simulink model "model1"  (R2021b)
settings: Solver=VariableStepAuto  StartTime=0.0  StopTime=10.0  RelTol=1e-3
values from neighbouring files (symbols this model uses):
  A = [   0    1 ... (first row only)    [config.m]
  A_m = [     0      1 ... (first row only)    [config.m]
  b = [0 ... (first row only)    [config.m]
  b_m = [0 ... (first row only)    [config.m]
  disturbance = 0    [config.m]    (also in task1.m = 1; task2.m = 1)
  gamma = 10000    [task1.m]    (also in task2.m = 100)
  k = b_0/a_m_0    (= 0.0434782608696)    [config.m]
  P = lyap(A_m', Q)    [config.m]
  x_0 = [1; 0]    [config.m]
settings Model: LastModifiedBy=popov
settings OptimizationCC: BlockReduction=off  BooleanDataType=off
settings DebuggingCC: SaveWithParameterizedLinksMsg=none  UnderspecifiedInitializationDetection=Classic  MergeDetectMultiDrivingBlocksExec=none  SignalResolutionControl=TryResolveAllWithWarning
settings HardwareCC: TargetUnknown=on
settings ModelReferenceCC: PropagateSignalLabelsOutOfModel=off

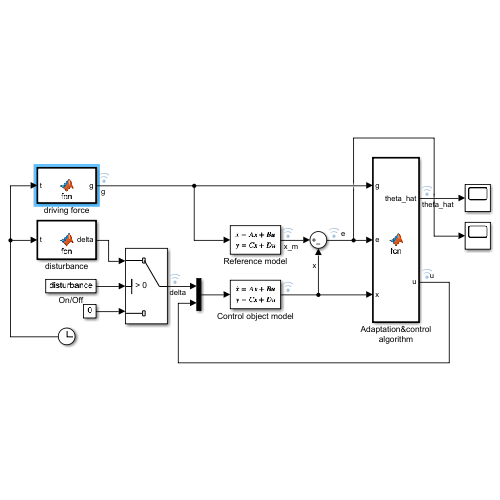
[thumbnail: Simulink's stored preview of the top-level diagram]
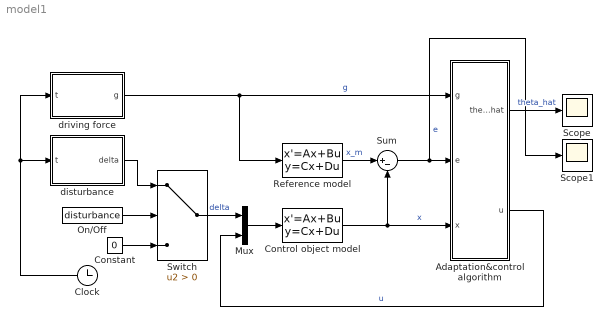
== system model1 ==
  Adaptation&control algorithm : MATLAB Function  TreatAsAtomicUnit=on
  Clock : Clock
  Constant : Constant  Value=0
  Control object model : StateSpace  A=A  B=[eye(2) b]  C=eye(2)  D=zeros(2,3)  InitialCondition=x_0
  Mux : Mux  Inputs=2
  On/Off : Constant  Value=disturbance
  Reference model : StateSpace  A=A_m  B=b_m  C=eye(2)  D=[0;0]  InitialCondition=0
  Scope : Scope
  Scope1 : Scope
  Sum : Sum  Inputs=|+-
  Switch : Switch  Criteria=u2 > Threshold
  disturbance : MATLAB Function  TreatAsAtomicUnit=on
  driving force : MATLAB Function  TreatAsAtomicUnit=on
  wires:
  Clock/1 -> disturbance/1(t), driving force/1(t)
  driving force/1(g) -> Reference model/1, Adaptation&control algorithm/1(g)  "g"
  Control object model/1 -> Sum/2, Adaptation&control algorithm/3(x)  "x"
  Sum/1 -> Scope1/1, Adaptation&control algorithm/2(e)  "e"
  Adaptation&control algorithm/2(u) -> Mux/2  "u"
  Reference model/1 -> Sum/1  "x_m"
  Mux/1 -> Control object model/1
  disturbance/1(delta) -> Switch/1
  Adaptation&control algorithm/1(theta_hat) -> Scope/1  "theta_hat"
  Constant/1 -> Switch/3
  Switch/1 -> Mux/1  "delta"
  On/Off/1 -> Switch/2

== matlab function model1/driving force ==
  data: t input; g output
function g = fcn(t)

g = 2*sign(sin(0.4*t)) + 3;

== matlab function model1/disturbance ==
  data: t input; delta output
function delta = fcn(t)

delta = [0.6*sin(10*t) + 0.1*sin(50*t);
        0.5*cos(12*t) + 0.2*sin(30*t)];

== matlab function model1/Adaptation&control algorithm ==
  data: theta_hat output; g input; e input; x input; u output; gamma parameter; b parameter; P parameter; k parameter
function [theta_hat, u]  = fcn(g, e, x, gamma, b, P, k)

theta_hat = gamma*x*b'*P*e;
u = theta_hat'*x + 1/k*g;
